simulink model "House_simple_spec"  (R2018b)
settings: Solver=ode45  StartTime=0  StopTime=365*24*3600  MaxStep=3600  RelTol=1e-3  EnableMultiTasking=on
InitFcn:
  | load('DE_TRY2010_04_averageYear')
undefined symbols (not defined in the file): delta_t_nom, dpcoeff, heatload, mass_times_cap, n_rad, path_carnot, Uground
libraries: carnot x9
settings Model: Creator=drhf  LastModifiedBy=drhf
settings DataIOCC: SaveFormat=Array  SignalLoggingSaveFormat=ModelDataLogs
settings OptimizationCC: ExpressionDepthLimit=2147483647  LifeSpan=inf
settings DebuggingCC: UnderspecifiedInitializationDetection=Classic  MergeDetectMultiDrivingBlocksExec=none  SolverPrmCheckMsg=warning  FcnCallInpInsideContextMsg=warning  StateNameClashWarn=warning  SFUnexpectedBacktrackingDiag=warning  SFNoUnconditionalDefaultTransitionDiag=warning  SFExecutionAtInitializationDiag=none
settings HardwareCC: ProdBitPerPointer=32  ProdBitPerSizeT=32  ProdBitPerPtrDiffT=32  ProdLargestAtomicFloat=None  ProdIntDivRoundTo=Undefined  ProdEndianess=Unspecified  ProdWordSize=32  ProdHWDeviceType=32-bit Generic
settings ModelReferenceCC: PropagateSignalLabelsOutOfModel=off
settings SFSimCC: SimUseLocalCustomCode=off
settings RTWCC: RTWUseLocalCustomCode=off
settings CodeAppCC: StateflowObjectComments=on
settings GRTTargetCC: TargetLangStandard=C89/C90 (ANSI)  GeneratePreprocessorConditionals=Disable all  CombineOutputUpdateFcns=off  GRTInterface=on
settings ConfigComp: CovMetricSettings=dw  CovHtmlReporting=on  CovSaveCumulativeToWorkspaceVar=on  CovSaveSingleToWorkspaceVar=on  CovExternalEMLEnable=off

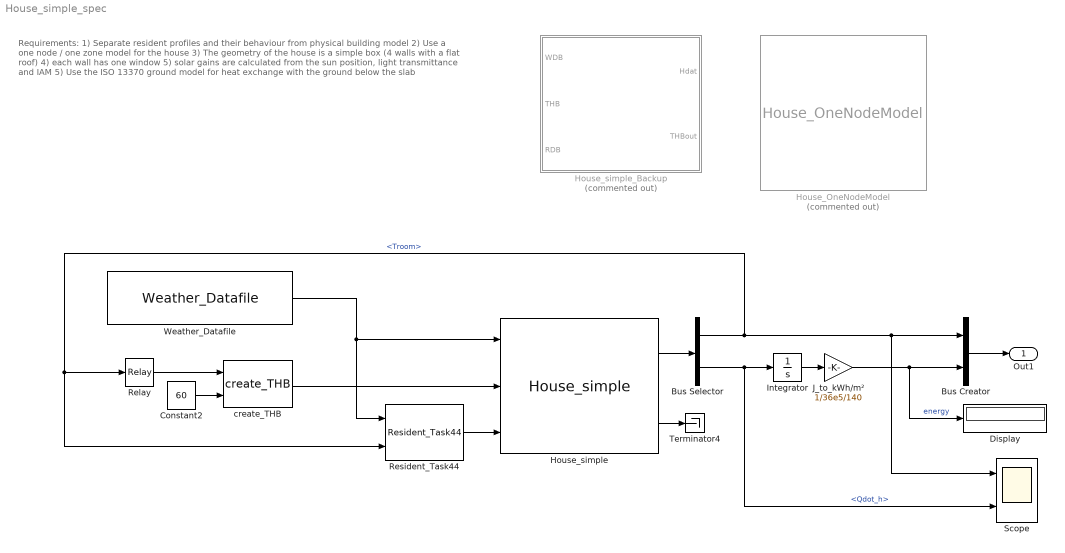
== system House_simple_spec ==
  note: Requirements:
      | 1) Separate resident profiles and their behaviour from physical building model
      | 2) Use a one node / one zone model for the house
      | 3) The geometry of the house is a simple box (4 walls with a flat roof)
      | 4) each wall has one window
      | 5) solar gains are calculated from the sun position, light transmittance and IAM
      | 5) Use the ISO 13370 ground model for heat exchange with the ground below the slab
  Bus Creator : BusCreator  Inputs=2
  Bus Selector : BusSelector  OutputSignals=Troom,Qdot.Qdot_h
  Constant2 : Constant  Value=60
  Display : Display
  House_OneNodeModel : carnot/Basic/Thermal_Models/House_OneNodeModel  Commented=on  A=140  UAout=0.197*(54.6+26.4)+0.286*((45.7+56.0)*2 -(12+4+3+4))  UAin=[1.5 1.5]  capa=0.5e6  tini=20  dtroom=inf  AziWin=[0 90 -180 -90]  Awin=[12 4 3 4]  Uwin="[1    1   1    1]*1.5"  Gwin="[1    1   1    1]*0.622*(1-0.15)"
  House_simple : carnot/Load/Houses/House_simple  tini=20  dtroom=inf  Tmeaninside=23.8  deltathetai=3.8  Tmeanoutside=11  deltathetae=9.3  tshift=319*3600  PathName=fullfile(path_carnot('libsl'), 'Load', 'Houses', 'House_simple', 'parameter_set')  FileName='Default_HouseSimple.mat'  userPath=off  userParam=off  Ahabit=140  Hroom=2.5  slabwidth=10  slablength=7  dwall=0.4  UAwall=100  capa=500000  utot=0.183  gammat=0  cond_ground=2  cp_ground=800  rho_ground=2500  Awindow=[12 4 3 4]  AziWin=[0 90 -180 -90]  Uwindow=[2 2 2 2]  Gwindow=[0.5 0.5 0.5 0.5]  alpha=10  H=1.2  W=1  Nwin=4  Ventilationrate=0.4  Heatrecovery=0  pnom=10000  dtnom=49.83  expo=1.3  mcap=10*4812  lin=100  qua=100
  House_simple_Backup : Subsystem  Commented=on  mask(House simple){tini=20, dtroom=inf, PathName=fullfile(path_carnot('libsl'),'Load','Houses','Simple_House_ISOgm_CONF','parameter_set'), FileName='<user defined>', userPath=off, userParam=on, Ahabit=140, Hroom=2.5, slabwidth=10, slablength=7, dwall=0.4, UAwall=100, capa=0.5e6, rtot=1/Uground, gammat=0, Tmeaninside=23.8, deltathetai=3.8, Tmeanoutside=11, deltathetae=9.3, tshift=319*3600, cond_ground=2.0, cp_ground=800, rho_ground=2500, Awindow=[12 4 3 4], AziWin=[0 90 -180 -90], Uwindow=[2 2 2 2], Gwindow=[0.5 0.5 0.5 0.5], alpha=10, H=1.2, W=1, Nwin=4, Ventilationrate=0.4, Heatrecovery=0, pnom=heatload, dtnom=delta_t_nom, expo=n_rad, mcap=mass_times_cap, lin=dpcoeff(1), qua=dpcoeff(2)}
      mask prompts: tini "Initial temperature in °C"; dtroom "Max. change of room temperature in K (standard value is 'inf')"; PathName "Path"; FileName "Parameter set"; userPath "Edit path and name of parameter set"; userParam "User defined parameters"; Ahabit "Heated living surface in m²"; Hroom "Height of rooms in m"; slabwidth "Width of slab in m"; slablength "Length of slab in m"; dwall "Average thickness of walls inlcuding insulation [m]"; UAwall "Total heat transfer to ambient (walls/roof) in W/K"; capa "Thermal capactiy per surface in J/m²/K"; rtot "total thermal resistance of slab (between Troom and Tground) [m²K/W]"; gammat "linear thermal transmittance associated with wall/floor junctions [W/mK]"; Tmeaninside "mean inside temperature over one year [°C]"; deltathetai "amplitude of monthly mean internal temperature [°C]"; Tmeanoutside "mean outside temperature over one year [°C]"; deltathetae "amplitude of monthly mean outside temperature [°C]"; tshift "time shift where external temperature sine-curve shows a mimimum [h]"; cond_ground "conductivity of ground [W/(m*K)]"; cp_ground "capacity of ground [J/(kg*K)]"; rho_ground "density of ground [kg/m^3]"; Awindow "Surface of 4 windows in m² (vector)"; AziWin "Orientation of the 4 windows (south 0, east -90,west 90)"; Uwindow "Heat loss coefficient 4 windows in W/m²/K [vector]"; Gwindow "Light transmittance 4 windows (0..1) * (1 - frame_part) [vector]"; alpha "Maximal opening angle in °"; H "Height of window opening in m"; W "Width of window opening in m"; Nwin "Number of windows for ventilation"; Ventilationrate "Ventilation rate in 1/h"; Heatrecovery "Heat recovery (0..1)"; pnom "Qdot_nom: nominal power in W"; dtnom "Tdiff_nom: nominal temperature difference in K"; expo "Radiator exponent (> 0)"; mcap "mass * capacity in J/K"; lin "l : linear pressure drop Pa/(kg/s)"; qua "q : quadratic pressure drop Pa/(kg/s)²"
      mask help:
      | Configurated building model, variables are defined in a mat-file (for example in "Default_SimpleHouseISOgm.mat") in the folder /parameter_set of the block.
      | Use of buttons in the "Picking a file" frame:
      | 1) "Carnot public data" choses a parameter file from the public data folder in Carnot. The "Path" is set to the public data folder.
      | 2) "Carnot internal data" choses a parameter file from the internal data folder in Carnot. The "Path" is set to the internal data folder.
      | 3) "From selected path" choses a parameter file from the "Path".
      | Allow editing "File" and "Path" with the checkbox. Be aware that the buttons in the "Picking a file" frame will anyway overwrite the edited values.
      mask init:
      | [ok, param] = CarnotCallbacks_SimpleHouseISOgmConf('SetParameters',gcbh,PathName,FileName);
      mask Help: web(fullfile(path_carnot('help'),'houseSimple.html'),'-helpbrowser')
      mask TypeOptions tini: House_OneNodeModel/tini | Radiator/tini
      mask TypeOptions dtroom: House_OneNodeModel/dtroom
      mask Callback userPath: [ok, param] = CarnotCallbacks_SimpleHouseISOgmConf('UserEdit',gcbh);
      mask Callback userParam: [ok, param] = CarnotCallbacks_SimpleHouseISOgmConf('UserEdit',gcbh);
      mask TypeOptions Ahabit: House_OneNodeModel/A | Ventilation/Ahabit
      mask TypeOptions Hroom: Simple_House_ISO_GroundModel/Hroom | Ventilation/Hroom
      mask TypeOptions slabwidth: HeatTransfer2Ground_ISO13370/slabwidth
      mask TypeOptions slablength: HeatTransfer2Ground_ISO13370/slablength
      mask TypeOptions dwall: HeatTransfer2Ground_ISO13370/dwall
      mask TypeOptions UAwall: House_OneNodeModel/UAout
      mask TypeOptions capa: House_OneNodeModel/capa
      mask TypeOptions rtot: HeatTransfer2Ground_ISO13370/rtot
      mask TypeOptions gammat: HeatTransfer2Ground_ISO13370/gammat
      mask TypeOptions Tmeaninside: HeatTransfer2Ground_ISO13370/Tmeaninside
      mask TypeOptions deltathetai: HeatTransfer2Ground_ISO13370/deltathetai
      mask TypeOptions Tmeanoutside: HeatTransfer2Ground_ISO13370/Tmeanoutside
      mask TypeOptions deltathetae: HeatTransfer2Ground_ISO13370/deltathetae
      mask TypeOptions tshift: HeatTransfer2Ground_ISO13370/tshift
      mask TypeOptions cond_ground: HeatTransfer2Ground_ISO13370/cond_ground
      mask TypeOptions cp_ground: HeatTransfer2Ground_ISO13370/cp_ground
      mask TypeOptions rho_ground: HeatTransfer2Ground_ISO13370/rho_ground
      mask TypeOptions Awindow: House_OneNodeModel/Awin
      mask TypeOptions AziWin: House_OneNodeModel/AziWin
      mask TypeOptions Uwindow: House_OneNodeModel/Uwin
      mask TypeOptions Gwindow: House_OneNodeModel/Gwin
      mask TypeOptions alpha: Ventilation/alpha
      mask TypeOptions H: Ventilation/H
      mask TypeOptions W: Ventilation/W
      mask TypeOptions Nwin: Ventilation/Nwin
      mask TypeOptions Ventilationrate: Ventilation/vent
      mask TypeOptions Heatrecovery: Ventilation/rec
      mask TypeOptions pnom: Radiator/pnom
      mask TypeOptions dtnom: Radiator/dtnom
      mask TypeOptions expo: Radiator/expo
      mask TypeOptions mcap: Radiator/mcap
      mask TypeOptions lin: Radiator/lin
      mask TypeOptions qua: Radiator/qua
      mask DialogControl Container10 Prompt: Calculation
      mask DialogControl ParameterGroupFile Prompt: Picking a parameter set
      mask DialogControl Control1 Prompt: Carnot public data
      mask DialogControl Control1 Callback: [ok, file] = CarnotCallbacks_SimpleHouseISOgmConf('GetFilename',gcbh, 'public');
      mask DialogControl Control3 Prompt: Carnot internal data
      mask DialogControl Control3 Callback: [ok, file] = CarnotCallbacks_SimpleHouseISOgmConf('GetFilename',gcbh, 'internal');
      mask DialogControl Control4 Prompt: Selected path
      mask DialogControl Control4 Callback: [ok, file] = CarnotCallbacks_SimpleHouseISOgmConf('GetFilename',gcbh, 'selected');
      mask DialogControl Container5 Prompt: House
      mask DialogControl Container13 Prompt: Ground
      mask DialogControl Container8 Prompt: Windows
      mask DialogControl Container9 Prompt: HVAC
      mask DialogControl Control5 Prompt: Save in Carnot internal data
      mask DialogControl Control5 Callback: [ok, param] = CarnotCallbacks_SimpleHouseISOgmConf('SaveFilename',gcbh, 'internal','SH');
      mask DialogControl Control6 Prompt: Save in selected path
      mask DialogControl Control6 Callback: [ok, param] = CarnotCallbacks_SimpleHouseISOgmConf('SaveFilename',gcbh, 'selected','SH');
      mask Display:
      | % user defined picture file
      | picfile = fullfile(path_carnot('intlibsl'), ...
      |         'Load','Houses','Simple_House_ISOgm_CONF','parameter_set', ...
      |         'Simple_House_ISOgm_CONF.jpg');
      | 
      | % show internal picture if defined
      | if ~BlockIsInCarnotLibrary ...      % if not located in library any more
      |         && exist(picfile,'file')    % AND picfile is present
      |     image(imread(picfile), [0.15 0.1 0.7 0.8])
      |     set_param(gcb, 'BackgroundColor', 'White')
      | else
      |     % show public picture
      |     plot([10,10,90,90,10]/120+0.1, [0,50,50,0,0]/100+0.1,...
      |          [100,60,40,0]/120+0.1,    [40,80,80,40]/100+0.1,...
      |          [20,34,34,20,20]/120+0.1, [40,40,20,20,40]/100+0.1,...
      |          [60,60,40,40]/120+0.1,    [0,40,40,0]/100+0.1,...
      |          [65,80,80,65,65]/120+0.1, [40,40,20,20,40]/100+0.1,...
      |          [47,54,54,47,47]/120+0.1, [35,35,4,4,35]/100+0.1,...
      |          [45,41]/120+0.1,          [20,20]/100+0.1)
      |      set_param(gcb, 'BackgroundColor', 'Orange')
      | end
  Integrator : Integrator
  J_to_kWh/m² : Gain  Gain=1/36e5/140
  Relay : Relay  OnSwitchValue=20.1  OffSwitchValue=19.9  OnOutputValue=0  OffOutputValue=800/3600
  Resident_Task44 : carnot/Load/Houses/Resident_Task44  period=24*3600  rep_seq_te=[0 1 6 7 8 9 11 12 13 18 19 20 22 23]*3600  rep_seq_de=[1 5 1 1 1 2 1 1 4 2 1 2 1 1]*3600  rep_seq_ye=[105 55 392.5 457.5 420 55 250 55 120 170 615 420 442.5 355]  rep_seq_to=[0 6 7 8 9 11 12 13 14 15 17 18 20 21 22]*3600  rep_seq_do=[6 1 1 1 2 1 1 1 1 2 1 2 1 1 2]*3600  rep_seq_yo=[4 2 3 2 0 1 3 2 1 0 1 2 4 3 4]*60  Topen=24  Tclose=23  TrAboveTa=2  TaTooCold=12  timeFIR=24  TaIni=12  starttime=8  stoptime=22  TroomShadeOn=23.8  TroomShadeOff=22.8  SolarShadeOn=300  SolarShadeOff=200  max_shade=1  CalcAirComp=off  mdotCO2=0  mdotH2O=0  mdotVOC=0
  Scope : Scope  NumInputPorts=2
  Terminator4 : Terminator
  Weather_Datafile : carnot/Weather/Weather_Datafile  PathName=path_carnot('data')  FileName='DE_TRY2010_04_averageYear.mat'  UserParam=off  VariableName=DE_TRY2010_04_averageYear  SampleTime=3600
  create_THB : carnot/Source/Simple/create_THB  p=1e5  fluid=Water  mix=0  mix2=0  mix3=0  dia=0.02  hgt=0  mID=No Pressure Drop
  Out1 : Outport
  wires:
  Weather_Datafile/1 -> Resident_Task44/1, House_simple/1
  Bus Creator/1 -> Out1/1
  House_simple/2 -> Terminator4/1
  House_simple/1 -> Bus Selector/1
  Bus Selector/1 -> Scope/1, Bus Creator/1, Resident_Task44/2, Relay/1  "<Troom>"
  Constant2/1 -> create_THB/2
  Relay/1 -> create_THB/1
  create_THB/1 -> House_simple/2
  Bus Selector/2 -> Scope/2, Integrator/1  "<Qdot_h>"
  Integrator/1 -> J_to_kWh/m²/1
  J_to_kWh/m²/1 -> Display/1, Bus Creator/2  "energy"
  Resident_Task44/1 -> House_simple/3

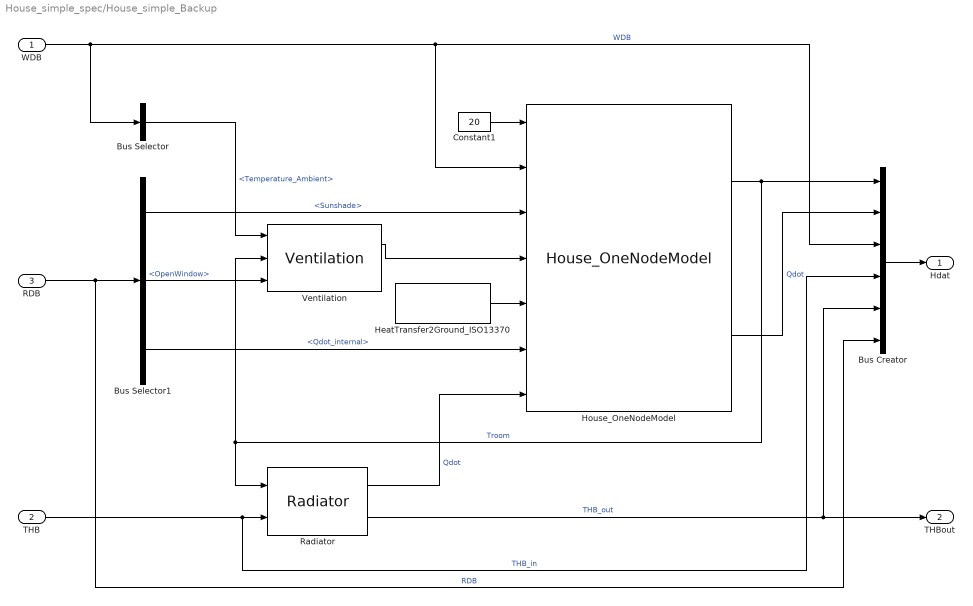
== system House_simple_spec/House_simple_Backup ==
  WDB : Inport
  THB : Inport  Port=2
  RDB : Inport  Port=3
  Bus Creator : BusCreator  Inputs=6
  Bus Selector : BusSelector  OutputSignals=Temperature_Ambient
  Bus Selector1 : BusSelector  OutputSignals=Sunshade,OpenWindow,Qdot_internal
  Constant1 : Constant  Value=20
  HeatTransfer2Ground_ISO13370 : carnot/Basic/Heat_Transfer/HeatTransfer2Ground_ISO13370  slabwidth=slabwidth  slablength=slablength  gammat=gammat  Tmeaninside=Tmeaninside  deltathetai=deltathetai  Tmeanoutside=Tmeanoutside  deltathetae=deltathetae  tshift=tshift  dwall=dwall  cond_ground=cond_ground  cp_ground=cp_ground  rho_ground=rho_ground  utot=0.183
  House_OneNodeModel : carnot/Basic/Thermal_Models/House_OneNodeModel  A=Ahabit  UAout=UAwall  UAin=UAneighbour  capa=capa  tini=tini  dtroom=dtroom  AziWin=AziWin  Awin=Awindow  Uwin=Uwindow  Gwin=Gwindow
  Radiator : carnot/Source/Heat_Exchanger/Radiator  pnom=pnom  dtnom=dtnom  expo=expo  mcap=mcap  tini=tini  lin=lin  qua=qua
  Ventilation : carnot/Source/Ventilation/Ventilation  Ahabit=Ahabit  Hroom=Hroom  vent=Ventilationrate  rec=Heatrecovery  ppmCO2=400  ppmVOC=0  alpha=alpha  H=H  W=W  Nwin=Nwin
  Hdat : Outport
  THBout : Outport  Port=2
  wires:
  WDB/1 -> Bus Selector/1, House_OneNodeModel/2, Bus Creator/3  "WDB"
  THB/1 -> Bus Creator/4, Radiator/2  "THB_in"
  Radiator/2 -> Bus Creator/5, THBout/1  "THB_out"
  House_OneNodeModel/1 -> Ventilation/2, Radiator/1, Bus Creator/1  "Troom"
  House_OneNodeModel/2 -> Bus Creator/2  "Qdot"
  Bus Creator/1 -> Hdat/1
  HeatTransfer2Ground_ISO13370/1 -> House_OneNodeModel/5
  Constant1/1 -> House_OneNodeModel/1
  Bus Selector1/3 -> House_OneNodeModel/6  "<Qdot_internal>"
  Radiator/1 -> House_OneNodeModel/7  "Qdot"
  Ventilation/1 -> House_OneNodeModel/4
  Bus Selector/1 -> Ventilation/1  "<Temperature_Ambient>"
  RDB/1 -> Bus Selector1/1, Bus Creator/6  "RDB"
  Bus Selector1/1 -> House_OneNodeModel/3  "<Sunshade>"
  Bus Selector1/2 -> Ventilation/3  "<OpenWindow>"
